simulink model "Sim3"  (R2024b)
settings: Solver=VariableStepAuto  StartTime=0.0  StopTime=10.0  RelTol=1e-3
undefined symbols (not defined in the file): A, B, c, K_m
settings Model: Creator=damor  LastModifiedBy=damor

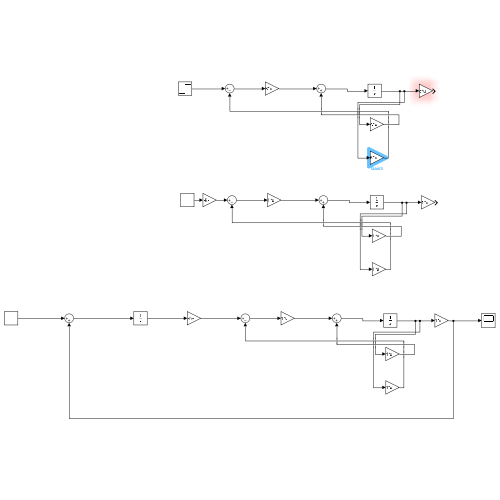
[thumbnail: Simulink's stored preview of the top-level diagram]
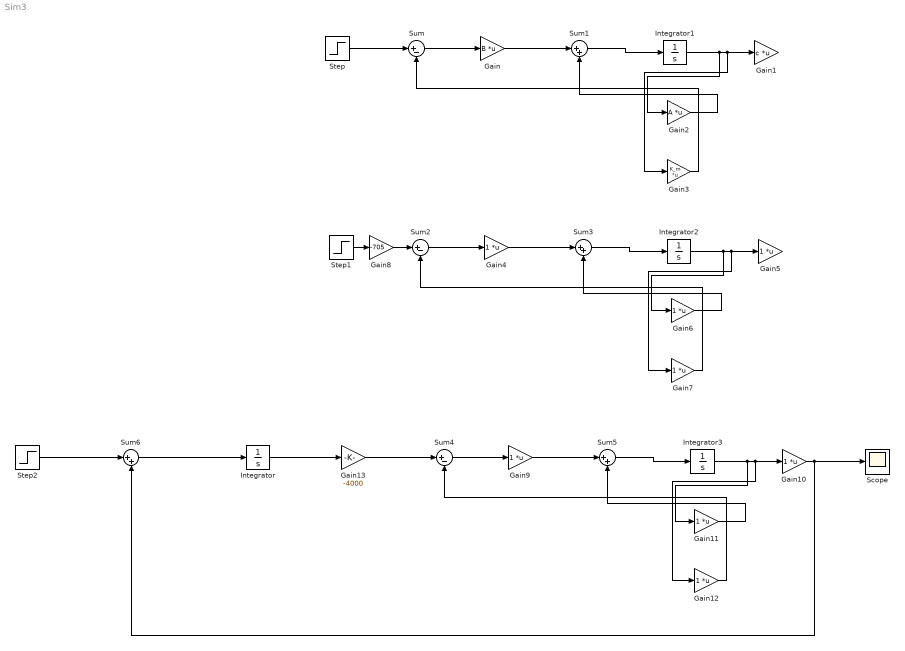
== system Sim3 ==
  Gain : Gain  Gain=B  Multiplication=Matrix(K*u)
  Gain1 : Gain  Gain=c  Multiplication=Matrix(K*u)
  Gain{4..7,9..12} (8 alike) : Gain  Multiplication=Matrix(K*u)
  Gain13 : Gain  Gain=-4000
  Gain2 : Gain  Gain=A  Multiplication=Matrix(K*u)
  Gain3 : Gain  Gain=K_m  Multiplication=Matrix(K*u)
  Gain8 : Gain  Gain=-705
  Integrator{,1..3} (4 alike) : Integrator
  Scope : Scope
  Step : Step  SampleTime=0
  Step1 : Step  SampleTime=0
  Step2 : Step  SampleTime=0
  Sum : Sum  Inputs=|+-
  Sum{1,3,5..6} (4 alike) : Sum  Inputs=|++
  Sum2 : Sum  Inputs=|+-
  Sum4 : Sum  Inputs=|+-
  wires:
  Sum/1 -> Gain/1
  Gain/1 -> Sum1/1
  Gain2/1 -> Sum1/2
  Integrator1/1 -> Gain2/1, Gain3/1, Gain1/1
  Sum1/1 -> Integrator1/1
  Gain3/1 -> Sum/2
  Step/1 -> Sum/1
  Step1/1 -> Gain8/1
  Gain7/1 -> Sum2/2
  Sum2/1 -> Gain4/1
  Gain6/1 -> Sum3/2
  Integrator2/1 -> Gain6/1, Gain7/1, Gain5/1
  Sum3/1 -> Integrator2/1
  Gain4/1 -> Sum3/1
  Gain8/1 -> Sum2/1
  Gain12/1 -> Sum4/2
  Sum4/1 -> Gain9/1
  Gain11/1 -> Sum5/2
  Integrator3/1 -> Gain11/1, Gain12/1, Gain10/1
  Sum5/1 -> Integrator3/1
  Gain9/1 -> Sum5/1
  Integrator/1 -> Gain13/1
  Gain13/1 -> Sum4/1
  Step2/1 -> Sum6/1
  Sum6/1 -> Integrator/1
  Gain10/1 -> Sum6/2, Scope/1
